simulink model "car_suspension_model"  (R2018b)
settings: Solver=VariableStepAuto  StartTime=0.0  StopTime=50  RelTol=1e-3
values from neighbouring files (symbols this model uses):
  b_car = 350    [suspension_system_parameters.m]
  b_wheel = 15000    [suspension_system_parameters.m]
  k_car = 80000    [suspension_system_parameters.m]
  k_wheel = 500000    [suspension_system_parameters.m]
  M_car = 3000    [suspension_system_parameters.m]
  W_mass = 350    [suspension_system_parameters.m]
settings Model: Creator=mayad  LastModifiedBy=mayad

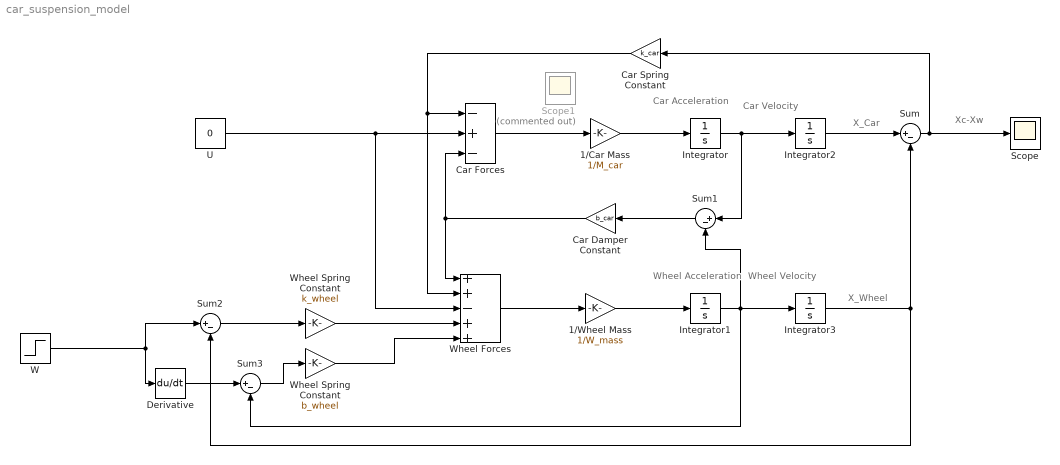
== system car_suspension_model ==
  note: Xc-Xw
  note: Car
      | Acceleration
  note: Wheel
      | Acceleration
  note: Car
      | Velocity
  note: Wheel
      | Velocity
  note: X_Car
  note: X_Wheel
  1/Car Mass : Gain  Gain=1/M_car
  1/Wheel Mass : Gain  Gain=1/W_mass
  "Car Damper Constant " : Gain  Gain=b_car
  Car Forces : Sum  Inputs=-+-
  "Car Spring Constant " : Gain  Gain=k_car
  Derivative : Derivative
  Integrator{,1..3} (4 alike) : Integrator
  Scope : Scope
  Scope1 : Scope  Commented=on
  Sum{,1..3} (4 alike) : Sum  Inputs=|+-
  U : Constant  Value=0  OutDataTypeStr=Inherit: Inherit via back propagation
  W : Step  SampleTime=0
  "Wheel Forces " : Sum  Inputs=++-++
  Wheel Spring Constant : Gain  Gain=b_wheel
  Wheel Spring Constant : Gain  Gain=k_wheel
  wires:
  Car Forces/1 -> 1/Car Mass/1
  "Wheel Forces "/1 -> 1/Wheel Mass/1
  1/Car Mass/1 -> Integrator/1
  1/Wheel Mass/1 -> Integrator1/1
  Integrator/1 -> Sum1/1, Integrator2/1
  Integrator1/1 -> Sum3/2, Sum1/2, Integrator3/1
  Integrator3/1 -> Sum2/2, Sum/2
  Integrator2/1 -> Sum/1
  Sum/1 -> Scope/1, "Car Spring Constant "/1
  "Car Spring Constant "/1 -> "Wheel Forces "/2, Car Forces/1
  Sum1/1 -> "Car Damper Constant "/1
  "Car Damper Constant "/1 -> "Wheel Forces "/1, Car Forces/3
  W/1 -> Sum2/1, Derivative/1
  Sum2/1 -> Wheel Spring Constant/1
  Derivative/1 -> Sum3/1
  Sum3/1 -> Wheel Spring Constant/1
  U/1 -> Car Forces/2, "Wheel Forces "/3
  Wheel Spring Constant/1 -> "Wheel Forces "/4
  Wheel Spring Constant/1 -> "Wheel Forces "/5
